simulink model "sensorCodeGenerationWrapper"  (R2022a)
settings: configuration reference "SensorCodeGenerationConfigurationSet" (kept outside this file)
model workspace (MAT data in the model file):
  SENSOR_PARAMETERS_NVM_ADDRESS_AS_UINT32 = Simulink.Parameter
  SENSOR_PARAMETERS_NVM_ADDRESS_AS_UINT32.Value = 1234
  SENSOR_PARAMETERS_NVM_ADDRESS_AS_UINT32.DataType = 'uint32'
  SENSOR_PARAMETERS_NVM_ADDRESS_AS_UINT32.Complexity = 'real'
  SENSOR_PARAMETERS_NVM_ADDRESS_AS_UINT32.Dimensions = [1 1]
settings Model: DataDictionary=sensorTargetSpecificData.sldd  EnableAccessToBaseWorkspace=off  Creator=The MathWorks, Inc.  LastModifiedBy=The MathWorks, Inc.
settings ConfigSetRef: SourceName=SensorCodeGenerationConfigurationSet

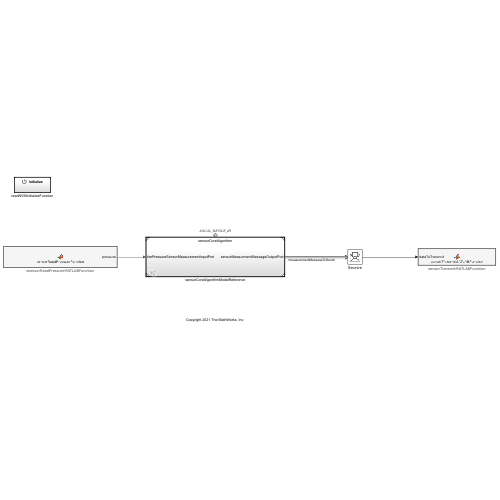
[thumbnail: Simulink's stored preview of the top-level diagram]
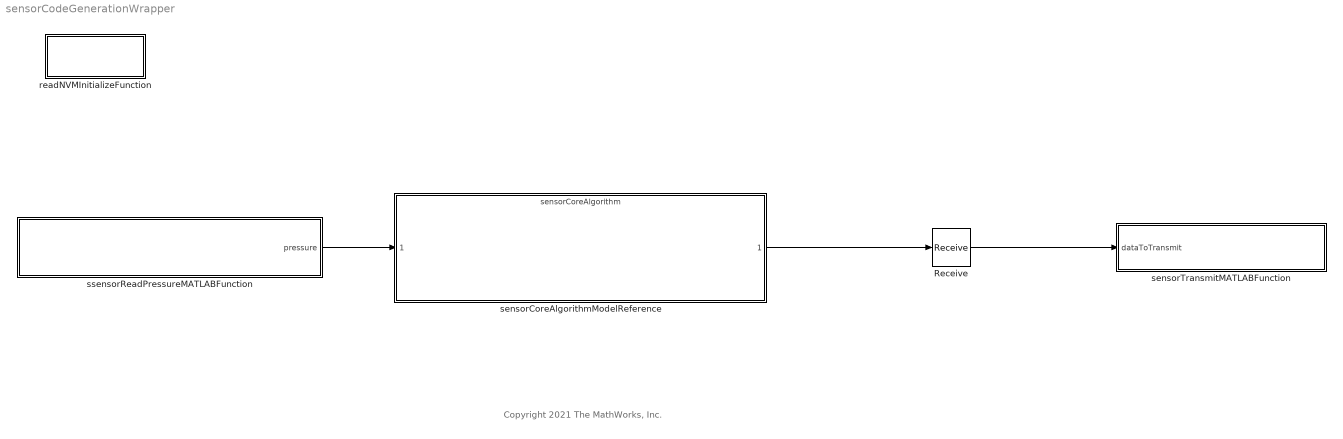
== system sensorCodeGenerationWrapper ==
  note: Copyright 2021 The MathWorks, Inc.
  Receive : Receive  InputPortMessageModes=m  UseInternalQueue=off  QueueOverwriting=on  QueueLength=1  QueueType=LIFO
  readNVMInitializeFunction : Subsystem  TreatAsAtomicUnit=on
  sensorCoreAlgorithmModelReference : ModelReference  OutputPortMessageModes=m  ModelNameDialog=sensorCoreAlgorithm  UsingDefaultArgumentValue=0  SimulationMode=Normal  ModelReferenceVersion=4.0
  sensorTransmitMATLABFunction : MATLAB Function  TreatAsAtomicUnit=on
  ssensorReadPressureMATLABFunction : MATLAB Function  TreatAsAtomicUnit=on
  wires:
  ssensorReadPressureMATLABFunction/1(pressure) -> sensorCoreAlgorithmModelReference/1
  sensorCoreAlgorithmModelReference/1 -> Receive/1
  Receive/1 -> sensorTransmitMATLABFunction/1(dataToTransmit)

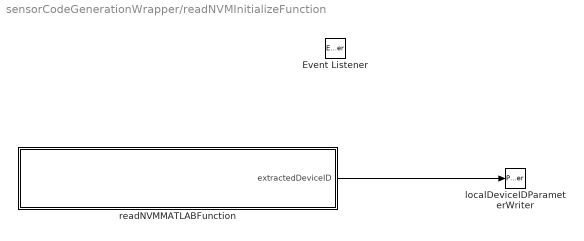
== system sensorCodeGenerationWrapper/readNVMInitializeFunction ==
  Event Listener : EventListener  DisableCoverage=on  EventName=reset
  localDeviceIDParameterWriter : ParameterWriter  ParameterOwnerBlock=../../sensorCoreAlgorithmModelReference  ParameterName=LOCAL_DEVICE_ID  ParameterInternalName=LOCAL_DEVICE_ID
  readNVMMATLABFunction : MATLAB Function  TreatAsAtomicUnit=on
  wires:
  readNVMMATLABFunction/1(extractedDeviceID) -> localDeviceIDParameterWriter/1

== matlab function sensorCodeGenerationWrapper/readNVMInitializeFunction/readNVMMATLABFunction ==
  data: extractedDeviceID output Bus: DeviceIDBusType; SENSOR_PARAMETERS_NVM_ADDRESS_AS_UINT32 parameter
function extractedDeviceID = readNVMMATLABFunction(SENSOR_PARAMETERS_NVM_ADDRESS_AS_UINT32) 

coder.extrinsic( 'warning' );

defaultDeviceID = deviceIDBusTypeDefaultConstructor( );

if( coder.target( 'Rtw' ) )
    
    extractedDeviceID = ...
        SensorTargetSpecificCodeExternalDependency.sensorReadNVMMatlabWrapper( SENSOR_PARAMETERS_NVM_ADDRESS_AS_UINT32, defaultDeviceID );
    
else
    warning( 'This block is only intended for code-generation.' );
    extractedDeviceID = defaultDeviceID;
end

return;

end

== matlab function sensorCodeGenerationWrapper/sensorTransmitMATLABFunction ==
  data: dataToTransmit input
function sensorTransmitMATLABFunction( dataToTransmit )

coder.extrinsic( 'warning' );

if( coder.target( 'Rtw' ) )
    
    SensorTargetSpecificCodeExternalDependency.sensorTransmitDataMATLABWrapper( dataToTransmit );
    
else
    warning( 'This block in only for code-generation.' );
end

return;

end

== matlab function sensorCodeGenerationWrapper/ssensorReadPressureMATLABFunction ==
  data: pressure output
function pressure   = sensorReadPressureFunction( ) 

coder.extrinsic( 'warning' );

pressure = double( 0 );

if( coder.target( 'Rtw' ) )

pressure = ...
    SensorTargetSpecificCodeExternalDependency.sensorReadPressureMATLABWrapper( );

else
    warning( 'This block is code-generation-only.' );
end

return;

end
